simulink model "Lab4_a"  (R2023b)
settings: Solver=VariableStepAuto  StartTime=0.0  StopTime=0.05  RelTol=1e-3
undefined symbols (not defined in the file or in its folder): Angle, Magnitude
libraries: spsVoltageMeasurementLib x6, spsCurrentMeasurementLib x4, spsSeriesRLCBranchLib x4, spsACVoltageSourceLib x2, spsLinearTransformerLib x2, sps_lib x1
settings Model: Creator=Shreetej  LastModifiedBy=Shreetej

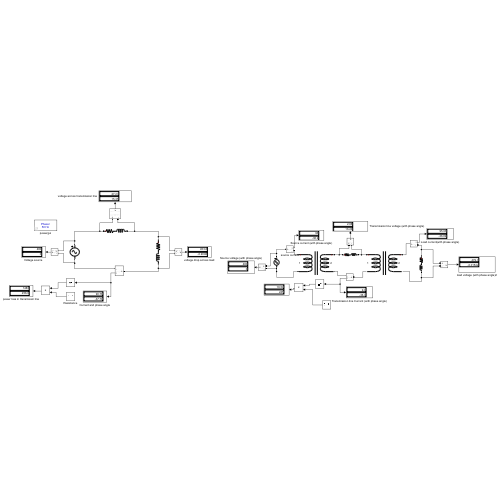
[thumbnail: Simulink's stored preview of the top-level diagram]
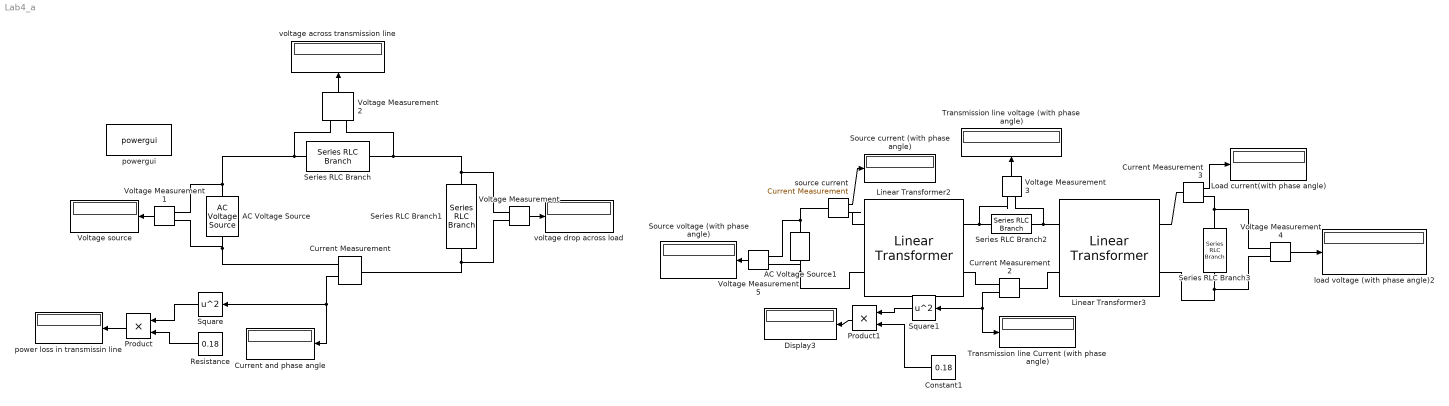
== system Lab4_a ==
  AC Voltage Source : spsACVoltageSourceLib/AC Voltage Source  Amplitude=480  Phase=0  Frequency=50  SampleTime=0  Measurements=None  BusType=swing  Pref=10e3  Qref=0  Qmin=-inf  Qmax=+inf
  AC Voltage Source1 : spsACVoltageSourceLib/AC Voltage Source  Amplitude=480  Phase=0  Frequency=50  SampleTime=0  Measurements=None  BusType=swing  Pref=10e3  Qref=0  Qmin=-inf  Qmax=+inf
  Constant1 : Constant  Value=0.18
  Current Measurement : spsCurrentMeasurementLib/Current Measurement  PhasorSimulation=on  OutputType=Magnitude-Angle  PSBequivalent=0
  Current Measurement2 : spsCurrentMeasurementLib/Current Measurement  PhasorSimulation=on  OutputType=Magnitude-Angle  PSBequivalent=0
  Current Measurement3 : spsCurrentMeasurementLib/Current Measurement  PhasorSimulation=on  OutputType=Magnitude-Angle  PSBequivalent=0
  Current and phase angle : Display
  Display3 : Display
  Linear Transformer2 : spsLinearTransformerLib/Linear Transformer  UNITS=SI  NominalPower=[ 250e6 60 ]  winding1=[480 0.000001 0.000001]  winding2=[4800 0.000001 0.000001]  ThreeWindings=off  winding3=[3.15e+05 0.7938 0.084225]  RmLm=[1.0804e+06 2866]  Measurements=None  DataType=on
  Linear Transformer3 : spsLinearTransformerLib/Linear Transformer  UNITS=SI  NominalPower=[ 250e6 60 ]  winding1=[4800 0.000001 0.000001]  winding2=[480 0.000001 0.000001]  ThreeWindings=off  winding3=[3.15e+05 0.7938 0.084225]  RmLm=[1.0804e+06 2866.1]  Measurements=None  DataType=on
  Load current(with phase angle) : Display
  Product : Product
  Product1 : Product
  Resistance : Constant  Value=0.18
  Series RLC Branch : spsSeriesRLCBranchLib/Series RLC Branch  LConnTagsString=__new0  RConnTagsString=__new0  BranchType=RL  Resistance=0.18  Inductance=0.0007639  SetiL0=off  InitialCurrent=0  Capacitance=1e-6  Setx0=off  InitialVoltage=0  Measurements=None
  Series RLC Branch1 : spsSeriesRLCBranchLib/Series RLC Branch  LConnTagsString=__new0  RConnTagsString=__new0  BranchType=RL  Resistance=4  Inductance=0.00955  SetiL0=off  InitialCurrent=0  Capacitance=1e-6  Setx0=off  InitialVoltage=0  Measurements=None
  Series RLC Branch2 : spsSeriesRLCBranchLib/Series RLC Branch  LConnTagsString=__new0  RConnTagsString=__new0  BranchType=RL  Resistance=0.18  Inductance=0.000764  SetiL0=off  InitialCurrent=0  Capacitance=1e-6  Setx0=off  InitialVoltage=0  Measurements=None
  Series RLC Branch3 : spsSeriesRLCBranchLib/Series RLC Branch  LConnTagsString=__new0  RConnTagsString=__new0  BranchType=RL  Resistance=4  Inductance=0.00955  SetiL0=off  InitialCurrent=0  Capacitance=1e-6  Setx0=off  InitialVoltage=0  Measurements=None
  Source current (with phase angle) : Display
  Source voltage (with phase angle) : Display
  Square : Math  Operator=square
  Square1 : Math  Operator=square
  Transmission line Current (with phase angle) : Display
  Transmission line voltage (with phase angle) : Display
  Voltage Measurement{,1..5} (6 alike) : spsVoltageMeasurementLib/Voltage Measurement  PhasorSimulation=on  OutputType=Magnitude-Angle  PSBequivalent=0
  "Voltage source " : Display
  load voltage (with phase angle)2 : Display
  power loss in transmissin line : Display
  powergui : sps_lib/powergui  Priority=1  SimulationMode=Phasor  SampleTime=50e-6  frequency=50  Iterations=50  frequencyindice=50  Pbase=100e6  ErrMax=1e-4  UnitsV=kV  UnitsW=MW  buscounter=0  FunctionMessages=off  echomessages=off  EnableUseOfTLC=off  CurrentSourceSwitches=off  DisableSnubberDevices=off  DisableRonSwitches=off  DisableVfSwitches=off  DisplayEquations=off  AutomaticDiscreteSolvers=off  SolverType=Tustin/Backward Euler (TBE)  Interpol=off  ExternalGateDelay=off  methode=off  Ts=100  x0status=blocks  SPID=on  SwTol=0  HookPort=off  NonlinearTolerance=1e-4  nMaxIteration=100  ContinueOnMaxIteration=off  RestoreLinks=warning  ResistiveCurrentMeasurement=off  Frange=[0:2:500]  Ylog=off  Xlog=on  ShowGrid=off  save=off  variable=ZData  structure=0  ZoomFFT=off  StartTime=0.0  cycles=1  DisplayStyle=1  fundamental=60  FreqAxis=off  MaxFrequency=1000  frequencyindicesteady=1  RmsSteady=1  display=off
  source current : spsCurrentMeasurementLib/Current Measurement  PhasorSimulation=on  OutputType=Magnitude-Angle  PSBequivalent=0
  voltage across transmission line : Display
  voltage drop across load : Display
  wires:
  Current Measurement/1 -> Square/1, Current and phase angle/1
  Voltage Measurement/1 -> voltage drop across load/1
  Voltage Measurement1/1 -> "Voltage source "/1
  Voltage Measurement2/1 -> voltage across transmission line/1
  Product/1 -> power loss in transmissin line/1
  Square/1 -> Product/1
  Resistance/1 -> Product/2
  source current/1 -> Source current (with phase angle)/1
  Current Measurement2/1 -> Transmission line Current (with phase angle)/1, Square1/1
  Current Measurement3/1 -> Load current(with phase angle)/1
  Square1/1 -> Product1/1
  Product1/1 -> Display3/1
  Voltage Measurement3/1 -> Transmission line voltage (with phase angle)/1
  Voltage Measurement4/1 -> load voltage (with phase angle)2/1
  Constant1/1 -> Product1/2
  Voltage Measurement5/1 -> Source voltage (with phase angle)/1
  connections:
  Series RLC Branch/RConn1 -- Voltage Measurement2/LConn2 -- Voltage Measurement/LConn1 -- Series RLC Branch1/LConn1
  Current Measurement/LConn1 -- Voltage Measurement/LConn2 -- Series RLC Branch1/RConn1
  AC Voltage Source/LConn1 -- Current Measurement/RConn1 -- Voltage Measurement1/LConn2
  AC Voltage Source/RConn1 -- Voltage Measurement1/LConn1 -- Voltage Measurement2/LConn1 -- Series RLC Branch/LConn1
  AC Voltage Source1/LConn1 -- Linear Transformer2/LConn2 -- Voltage Measurement5/LConn2
  Series RLC Branch2/RConn1 -- Voltage Measurement3/LConn2 -- Linear Transformer3/LConn1
  Series RLC Branch2/LConn1 -- Voltage Measurement3/LConn1 -- Linear Transformer2/RConn1
  Linear Transformer3/RConn2 -- Voltage Measurement4/LConn2 -- Series RLC Branch3/RConn1
  AC Voltage Source1/RConn1 -- Voltage Measurement5/LConn1 -- source current/LConn1
  source current/RConn1 -- Linear Transformer2/LConn1
  Current Measurement2/LConn1 -- Linear Transformer3/LConn2
  Linear Transformer2/RConn2 -- Current Measurement2/RConn1
  Linear Transformer3/RConn1 -- Current Measurement3/LConn1
  Current Measurement3/RConn1 -- Voltage Measurement4/LConn1 -- Series RLC Branch3/LConn1
